simulink model "ControlLoopSimKoopman"  (R2018b)
settings: Solver=FixedStepAuto  StartTime=0.0  StopTime=Tsim  FixedStep=Ts  RelTol=1e-3
values from neighbouring files (symbols this model uses):
  Ts = 0.01    [simulation.m]    (also in simulationKoop.m)
  x0 = [80/3.6; 0; -5/180*pi]    [simulation.m]    (also in simulationKoop.m = [60/3.6; 0; -5/180*pi])
undefined symbols (not defined in the file or in its folder): nRef, nSignal, reference, steering, TransformInputs
settings Model: Creator=Marko  LastModifiedBy=Marko

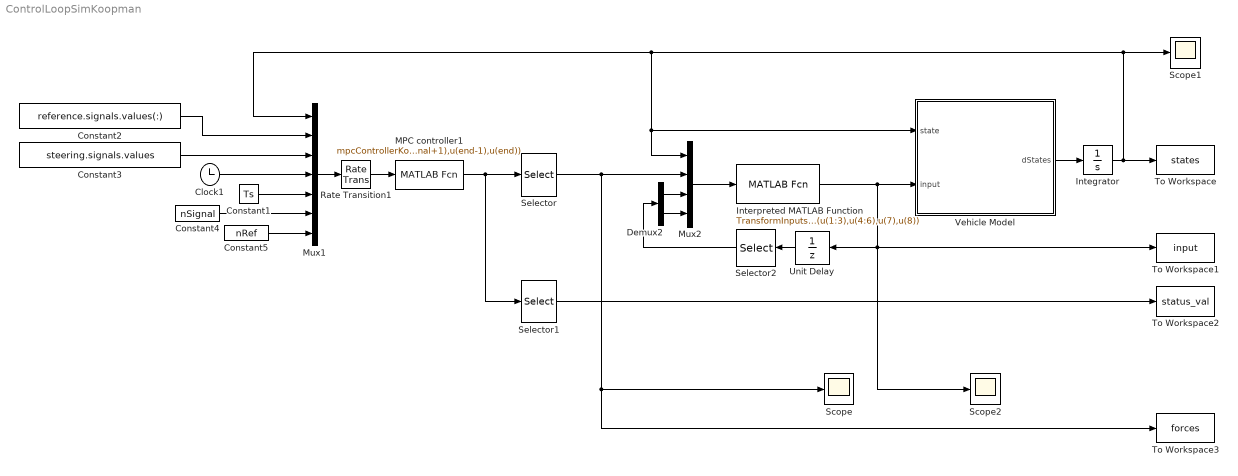
== system ControlLoopSimKoopman ==
  Clock1 : Clock
  Constant1 : Constant  Value=Ts
  Constant2 : Constant  Value=reference.signals.values(:)  SampleTime=Ts
  Constant3 : Constant  Value=steering.signals.values  SampleTime=Ts
  Constant4 : Constant  Value=nSignal
  Constant5 : Constant  Value=nRef
  Demux2 : Demux  Outputs=2
  Integrator : Integrator  InitialCondition=x0
  Interpreted MATLAB Function : MATLABFcn  MATLABFcn=TransformInputs(u(1:3),u(4:6),u(7),u(8))  OutputDimensions=3
  MPC controller1 : MATLABFcn  MATLABFcn=mpcControllerKoop(u(1:3), u(4:4+nSignal*nRef-1), u(4+nSignal*nRef:4+nSignal*nRef+nSignal-1), u(4+nSignal*nRef+nSignal),u(4+nSignal*nRef+nSignal+1),u(end-1),u(end))  OutputDimensions=3 + 1
  Mux1 : Mux  Inputs=7
  Mux2 : Mux
  Rate Transition1 : RateTransition  OutPortSampleTime=Ts
  Scope : Scope
  Scope1 : Scope
  Scope2 : Scope
  Selector : Selector  InputPortWidth=4  IndexOptions=Index vector (dialog)  Indices=[1 2 3]  OutputSizes=1
  Selector1 : Selector  InputPortWidth=4  IndexOptions=Index vector (dialog)  Indices=4  OutputSizes=1
  Selector2 : Selector  InputPortWidth=3  IndexOptions=Index vector (dialog)  Indices=[1 2]  OutputSizes=1
  To Workspace : ToWorkspace  VariableName=states  SaveFormat=Structure With Time  SampleTime=Ts
  To Workspace1 : ToWorkspace  VariableName=input  SaveFormat=Structure With Time  SampleTime=Ts
  To Workspace2 : ToWorkspace  VariableName=status_val  SaveFormat=Structure With Time  SampleTime=Ts
  To Workspace3 : ToWorkspace  VariableName=forces  SaveFormat=Structure With Time  SampleTime=Ts
  Unit Delay : UnitDelay  InitialCondition=[0; 0; 0]  SampleTime=Ts
  Vehicle Model : MATLAB Function  TreatAsAtomicUnit=on
  wires:
  Vehicle Model/1(dStates) -> Integrator/1
  Selector1/1 -> To Workspace2/1
  Selector/1 -> To Workspace3/1, Scope/1, Mux2/2
  Demux2/1 -> Mux2/3
  Mux2/1 -> Interpreted MATLAB Function/1
  Selector2/1 -> Demux2/1
  Unit Delay/1 -> Selector2/1
  Interpreted MATLAB Function/1 -> Scope2/1, To Workspace1/1, Unit Delay/1, Vehicle Model/2(input)
  Demux2/2 -> Mux2/4
  Constant4/1 -> Mux1/6
  Constant2/1 -> Mux1/2
  Constant1/1 -> Mux1/5
  Constant5/1 -> Mux1/7
  Rate Transition1/1 -> MPC controller1/1
  Mux1/1 -> Rate Transition1/1
  Constant3/1 -> Mux1/3
  Integrator/1 -> Scope1/1, Mux1/1, Mux2/1, Vehicle Model/1(state), To Workspace/1
  Clock1/1 -> Mux1/4
  MPC controller1/1 -> Selector1/1, Selector/1

== matlab function ControlLoopSimKoopman/Vehicle Model ==
  data: state input; dStates output; input input
function dStates  = BicycleModel(state,input)

% Extract states
vx = state(1);
vy = state(2);
yawRate = state(3);

% Extract inputs
deltaF = input(1);
sF = input(2);
sR = input(3);

% Load parameters
vehicle = LoadVehicleParameters();

% Vehicle parameters
a = vehicle.a;
b = vehicle.b;
m = vehicle.Mass;
I = vehicle.Izz;

% Air drag parameters
cw = vehicle.cw;
rho = vehicle.rho;
Aw = vehicle.Aw;

% Tyre parameters
Cxf = vehicle.Cxf;
Cyf = vehicle.Cyf;
Cxr = vehicle.Cxr;
Cyr = vehicle.Cyr;

% Lateral velocities
vyf = vy + a*yawRate;
vyr = vy - b*yawRate;
% Longitudinal velocities
vxf = vx;
vxr = vx;

% TYRE VELOCITIES
% Cornering velocities
vcf = vyf*cos(deltaF) - vxf*sin(deltaF);
vcr = vyr;
% Longitudinal velocities
vlf = vyf*sin(deltaF) + vxf*cos(deltaF);
vlr = vxr;

% TYRE SLIP ANGLES
alpha_f = atan2(vcf,vlf);
alpha_r = atan2(vcr,vlr);

% Longitudinal and cornering forces
Flf = Cxf*sF;
Flr = Cxr*sR;
Fcf = -Cyf*alpha_f;
Fcr = -Cyr*alpha_r;

% AXLE FORCES
% Lateral forces
Fyf = Flf*sin(deltaF) + Fcf*cos(deltaF);
Fyr = Fcr;
% Longitudinal forces
Fxf = Flf*cos(deltaF) - Fcf*sin(deltaF);
Fxr = Flr;

dVx = 1/m * (m*yawRate*vy - 0.5*cw*rho*Aw*sqrt(vx^2+vy^2)*vx + Fxf + Fxr);
dVy = 1/m * (-m*yawRate*vx - 0.5*cw*rho*Aw*sqrt(vx^2+vy^2)*vy + Fyf + Fyr);
dYawRate = 1/I * (Fyf*a - Fyr*b);

dStates = [dVx; dVy; dYawRate];

end
